simulink model "untitled2"  (R2016a)
settings: Solver=VariableStepAuto  StartTime=0.0  StopTime=5  RelTol=1e-3
libraries: SimscapeMacros x14, elec_lib x7, ProjectBlocks x5, fl_lib x3, simulink x2, simulink_extras x1, nesl_utility x1
settings Model: Creator=Peter  LastModifiedBy=Peter

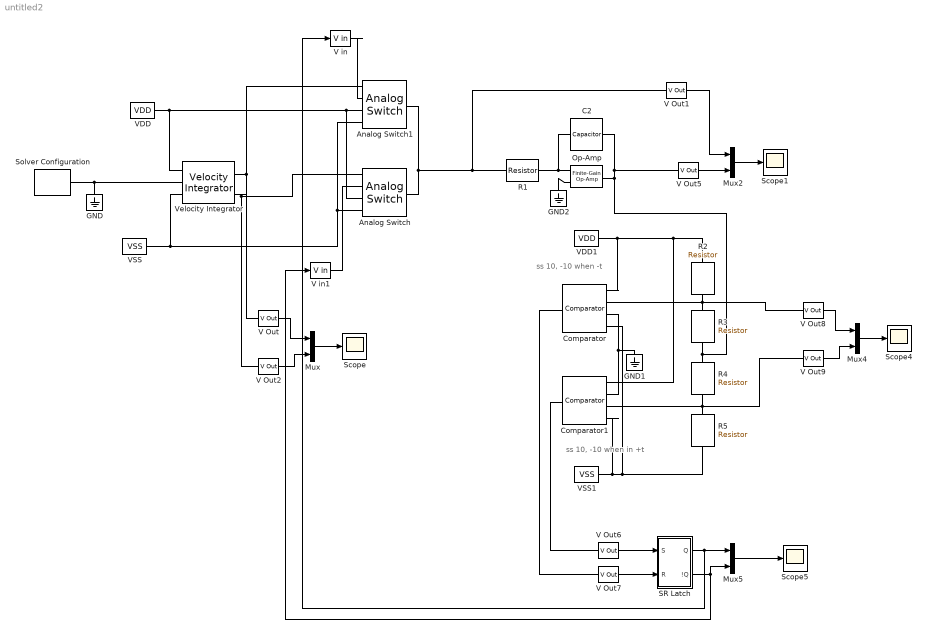
== system untitled2 ==
  note: ss 10, -10 when -t
  note: ss 10, -10 when in +t
  Analog Switch : ProjectBlocks/Analog Switch
  Analog Switch1 : ProjectBlocks/Analog Switch
  C2 : elec_lib/Passive Devices/Capacitor  enable_table=0  c=1e-6 F  Cvec=[ 1e-5 1e-6 ] F  Vvec=[ 0 10 ] V  CV_table_symmetry=1  C_tol=5  enable_C_tol=0  tol_distribution=1  nSigma=4  r=1e-6 Ohm  g=0 1/Ohm  initV=0 V  enable_operating_limits=0  operating_limit_action=2  max_working_voltage_range=[ -25 25 ] V  power_rating=1 W  enable_faults=0  fault_action=1  Cscale_faulted=100  R_faulted=0.001 Ohm  G_faulted=0 1/Ohm  tau_fault=0.001 s  enable_temporal_fault=0  t_fault=1 s  enable_behavioral_fault=0  max_permissible_voltage_range=[ -100 100 ] V  t_fail_on_voltage=1 s
  Comparator : ProjectBlocks/Comparator
  Comparator1 : ProjectBlocks/Comparator
  GND : fl_lib/Electrical/Electrical Elements/Electrical Reference
  GND1 : fl_lib/Electrical/Electrical Elements/Electrical Reference
  GND2 : fl_lib/Electrical/Electrical Elements/Electrical Reference
  Mux{,2,4..5} (4 alike) : Mux  Inputs=2
  Op-Amp : elec_lib/Integrated Circuits/Finite-Gain Op-Amp  A=1000  Rin=1e6 Ohm  Rout=100 Ohm  Vmin=-10 V  Vmax=10 V
  R1 : elec_lib/Passive Devices/Resistor  R=100e3 Ohm  R_tol=5  enable_R_tol=0  tol_distribution=1  nSigma=4  enable_operating_limits=0  operating_limit_action=2  max_working_voltage=100 V  power_rating=1 W  enable_faults=0  fault_action=1  R_faulted=Inf Ohm  enable_temporal_fault=0  t_fault=1 s  enable_behavioral_fault=0  max_permissible_current=1 A  t_fail_on_current=1 s  noise_mode=0  sample_time=0.001 s  repeatability=1  auto_seed=2499412182  user_seed=0  Tdevice=25 degC  alpha=0.00393 1/K  Tmeas=25 degC  thermal_mass=100 J/K  initial_temperature=25 degC  power_derating_T1=70 degC  power_derating_T2=155 degC  operating_temperature_range_vec=[ -50 150 ] degC
  R2 : elec_lib/Passive Devices/Resistor  R=10e3 Ohm  R_tol=5  enable_R_tol=0  tol_distribution=1  nSigma=4  enable_operating_limits=0  operating_limit_action=2  max_working_voltage=100 V  power_rating=1 W  enable_faults=0  fault_action=1  R_faulted=Inf Ohm  enable_temporal_fault=0  t_fault=1 s  enable_behavioral_fault=0  max_permissible_current=1 A  t_fail_on_current=1 s  noise_mode=0  sample_time=0.001 s  repeatability=1  auto_seed=1657856668  user_seed=0  Tdevice=25 degC  alpha=0.00393 1/K  Tmeas=25 degC  thermal_mass=100 J/K  initial_temperature=25 degC  power_derating_T1=70 degC  power_derating_T2=155 degC  operating_temperature_range_vec=[ -50 150 ] degC
  R3 : elec_lib/Passive Devices/Resistor  R=5e3 Ohm  R_tol=5  enable_R_tol=0  tol_distribution=1  nSigma=4  enable_operating_limits=0  operating_limit_action=2  max_working_voltage=100 V  power_rating=1 W  enable_faults=0  fault_action=1  R_faulted=Inf Ohm  enable_temporal_fault=0  t_fault=1 s  enable_behavioral_fault=0  max_permissible_current=1 A  t_fail_on_current=1 s  noise_mode=0  sample_time=0.001 s  repeatability=1  auto_seed=2534392050  user_seed=0  Tdevice=25 degC  alpha=0.00393 1/K  Tmeas=25 degC  thermal_mass=100 J/K  initial_temperature=25 degC  power_derating_T1=70 degC  power_derating_T2=155 degC  operating_temperature_range_vec=[ -50 150 ] degC
  R4 : elec_lib/Passive Devices/Resistor  R=5e3 Ohm  R_tol=5  enable_R_tol=0  tol_distribution=1  nSigma=4  enable_operating_limits=0  operating_limit_action=2  max_working_voltage=100 V  power_rating=1 W  enable_faults=0  fault_action=1  R_faulted=Inf Ohm  enable_temporal_fault=0  t_fault=1 s  enable_behavioral_fault=0  max_permissible_current=1 A  t_fail_on_current=1 s  noise_mode=0  sample_time=0.001 s  repeatability=1  auto_seed=906187493  user_seed=0  Tdevice=25 degC  alpha=0.00393 1/K  Tmeas=25 degC  thermal_mass=100 J/K  initial_temperature=25 degC  power_derating_T1=70 degC  power_derating_T2=155 degC  operating_temperature_range_vec=[ -50 150 ] degC
  R5 : elec_lib/Passive Devices/Resistor  R=10e3 Ohm  R_tol=5  enable_R_tol=0  tol_distribution=1  nSigma=4  enable_operating_limits=0  operating_limit_action=2  max_working_voltage=100 V  power_rating=1 W  enable_faults=0  fault_action=1  R_faulted=Inf Ohm  enable_temporal_fault=0  t_fault=1 s  enable_behavioral_fault=0  max_permissible_current=1 A  t_fail_on_current=1 s  noise_mode=0  sample_time=0.001 s  repeatability=1  auto_seed=749100358  user_seed=0  Tdevice=25 degC  alpha=0.00393 1/K  Tmeas=25 degC  thermal_mass=100 J/K  initial_temperature=25 degC  power_derating_T1=70 degC  power_derating_T2=155 degC  operating_temperature_range_vec=[ -50 150 ] degC
  SR Latch : Subsystem
  Scope{,1,4..5} (4 alike) : Scope
  Solver Configuration : nesl_utility/Solver Configuration  PhysicalDomain=network_engine_domain  SubClassName=solver  LeftPortType=input  RightPortType=generic  Accelerate=off  Tones=[]  Harmonics=[]  SimulateNoise=off  Profile=off  UseLocalSampling=off  EnableSwitchedLinearOptims=on  FrequencyDomain=off  UseCCode=off  RelTol=0.001  AbsTol=1e-06  MinStep=1e-09  ToWorkspace=off  RevertToSquareIcSolve=off  NumHomotopyIterations=100  PhasorMode=off  PhasorModeNumHarmonics=1  OverrideAbsTol=off  DoDC=off  ResidualTolerance=1e-09  UseLocalSolver=off  LocalSolverChoice=NE_BACKWARD_EULER_ADVANCER  LocalSolverSampleTime=0.001  DoFixedCost=off  MaxNonlinIter=3  MaxModeIter=2  LinearAlgebra=Sparse  DelaysMemoryBudget=1024  AutomaticFiltering=on  FilteringTimeConstant=0.001
  V Out{,1..2,5..9} (8 alike) : SimscapeMacros/V Out
  V in : SimscapeMacros/V in
  V in1 : SimscapeMacros/V in
  VDD : SimscapeMacros/VDD
  VDD1 : SimscapeMacros/VDD
  VSS : SimscapeMacros/VSS
  VSS1 : SimscapeMacros/VSS
  Velocity Integrator : ProjectBlocks/Velocity Integrator
  wires:
  Mux/1 -> Scope/1
  V Out/1 -> Mux/1
  V Out2/1 -> Mux/2
  Mux2/1 -> Scope1/1
  V Out5/1 -> Mux2/2
  V Out1/1 -> Mux2/1
  V Out7/1 -> SR Latch/2(R)
  Mux4/1 -> Scope4/1
  V Out8/1 -> Mux4/1
  V Out9/1 -> Mux4/2
  Mux5/1 -> Scope5/1
  V Out6/1 -> SR Latch/1(S)
  SR Latch/1(Q) -> V in/1, Mux5/1
  SR Latch/2(!Q) -> Mux5/2, V in1/1
  connections:
  GND/LConn1 -- Velocity Integrator/LConn2 -- Solver Configuration/RConn1
  Velocity Integrator/RConn1 -- V Out/LConn1 -- Analog Switch1/LConn1
  Velocity Integrator/LConn1 -- Analog Switch/LConn3 -- Analog Switch1/LConn3 -- VDD/RConn1
  Velocity Integrator/LConn3 -- Analog Switch1/LConn4 -- Analog Switch/LConn4 -- VSS/RConn1
  Velocity Integrator/RConn2 -- Analog Switch/LConn1 -- V Out2/LConn1
  Analog Switch/RConn1 -- V Out1/LConn1 -- R1/LConn1 -- Analog Switch1/RConn1
  Op-Amp/LConn2 -- C2/RConn1 -- R1/RConn1
  C2/LConn1 -- V Out5/LConn1 -- R4/LConn1 -- R3/RConn1 -- Op-Amp/RConn1
  GND2/LConn1 -- Op-Amp/LConn1
  Comparator/LConn3 -- Comparator1/LConn2 -- GND1/LConn1
  R3/LConn1 -- V Out8/LConn1 -- Comparator/LConn2 -- R2/RConn1
  R5/LConn1 -- V Out9/LConn1 -- Comparator1/LConn3 -- R4/RConn1
  VSS1/RConn1 -- Comparator1/LConn4 -- R5/RConn1 -- Comparator/LConn4
  VDD1/RConn1 -- Comparator/LConn1 -- Comparator1/LConn1 -- R2/LConn1
  V Out6/LConn1 -- Comparator1/RConn1
  V Out7/LConn1 -- Comparator/RConn1
  V in/RConn1 -- Analog Switch1/LConn2
  V in1/RConn1 -- Analog Switch/LConn2

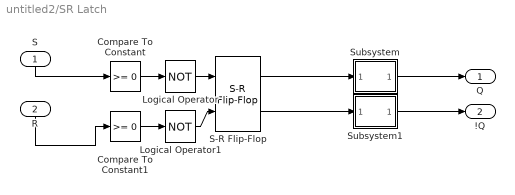
== system untitled2/SR Latch ==
  S : Inport
  R : Inport  Port=2
  Compare To Constant : simulink/Logic and Bit Operations/Compare To Constant  relop=>=  const=0  OutDataTypeStr=boolean
  Compare To Constant1 : simulink/Logic and Bit Operations/Compare To Constant  relop=>=  const=0  OutDataTypeStr=boolean
  Logical Operator : Logic  Operator=NOT  AllPortsSameDT=off  OutDataTypeStr=boolean
  Logical Operator1 : Logic  Operator=NOT  AllPortsSameDT=off  OutDataTypeStr=boolean
  S-R Flip-Flop : simulink_extras/Flip Flops/S-R Flip-Flop  initial_condition=1
  Subsystem : Subsystem
  Subsystem1 : Subsystem
  Q : Outport
  !Q : Outport  Port=2
  wires:
  Logical Operator1/1 -> S-R Flip-Flop/2
  Logical Operator/1 -> S-R Flip-Flop/1
  S/1 -> Compare To Constant/1
  R/1 -> Compare To Constant1/1
  Compare To Constant1/1 -> Logical Operator1/1
  S-R Flip-Flop/2 -> Subsystem1/1(In1)
  Compare To Constant/1 -> Logical Operator/1
  Subsystem1/1(Out1) -> !Q/1
  Subsystem/1(Out1) -> Q/1
  S-R Flip-Flop/1 -> Subsystem/1(In1)

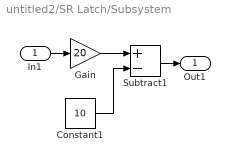
== system untitled2/SR Latch/Subsystem ==
  In1 : Inport
  Constant1 : Constant  Value=10
  Gain : Gain  Gain=20
  Subtract1 : Sum  Inputs=+-
  Out1 : Outport
  wires:
  Gain/1 -> Subtract1/1
  Constant1/1 -> Subtract1/2
  In1/1 -> Gain/1
  Subtract1/1 -> Out1/1

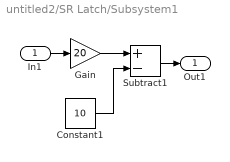
== system untitled2/SR Latch/Subsystem1 ==
  In1 : Inport
  Constant1 : Constant  Value=10
  Gain : Gain  Gain=20
  Subtract1 : Sum  Inputs=+-
  Out1 : Outport
  wires:
  Gain/1 -> Subtract1/1
  Constant1/1 -> Subtract1/2
  In1/1 -> Gain/1
  Subtract1/1 -> Out1/1
